simulink model "wetmodel_basic"  (R2020b)
settings: Solver=ode45  StartTime=0.0  StopTime=inf  RelTol=1e-3  EnableMultiTasking=on
libraries: dsparch4 x3, robotlib x1, dspsigops x1
settings Model: Tag=MP_system  EnablePacing=on  Creator=Andries  LastModifiedBy=LocalAdmin
settings DataIOCC: LimitDataPoints=on  SaveFormat=Array  SignalLoggingSaveFormat=ModelDataLogs  ReturnWorkspaceOutputs=off
settings OptimizationCC: ExpressionDepthLimit=2147483647  LifeSpan=inf
settings DebuggingCC: UnderspecifiedInitializationDetection=Classic  MergeDetectMultiDrivingBlocksExec=none  SolverPrmCheckMsg=warning  FcnCallInpInsideContextMsg=warning  StateNameClashWarn=warning  SFUnexpectedBacktrackingDiag=warning  SFNoUnconditionalDefaultTransitionDiag=warning  SFExecutionAtInitializationDiag=none  ArithmeticOperatorsInVariantConditions=warning
settings HardwareCC: ProdBitPerPointer=32  ProdBitPerSizeT=32  ProdBitPerPtrDiffT=32  ProdLargestAtomicFloat=None  ProdIntDivRoundTo=Undefined  ProdEndianess=Unspecified  ProdWordSize=32  ProdHWDeviceType=32-bit Generic
settings ModelReferenceCC: PropagateSignalLabelsOutOfModel=off
settings SFSimCC: SimUseLocalCustomCode=off  CustomCodeUndefinedFunction=UseInterfaceOnly
settings RTWCC: RTWUseLocalCustomCode=off
settings CodeAppCC: StateflowObjectComments=on
settings GRTTargetCC: TargetLangStandard=C89/C90 (ANSI)  CombineOutputUpdateFcns=off  GRTInterface=on
settings ConfigComp: CovMetricSettings=dw  CovSaveCumulativeToWorkspaceVar=on  CovSaveSingleToWorkspaceVar=on  CovExternalEMLEnable=off

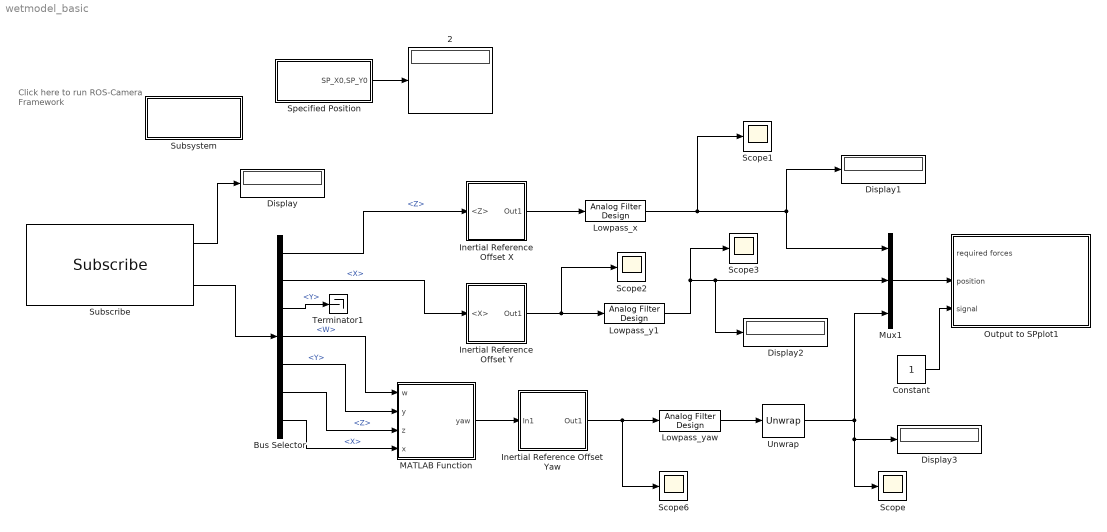
== system wetmodel_basic ==
  note: Click here to run
      | ROS-Camera Framework
  "  2" : Display
  Bus Selector : BusSelector  OutputSignals=Pose.Position.Z,Pose.Position.X,Pose.Position.Y,Pose.Orientation.W,Pose.Orientation.Y,Pose.Orientation.Z,Pose.Orientation.X
  Constant : Constant
  Display{,1..3} (4 alike) : Display
  Inertial Reference Offset X : Subsystem
  Inertial Reference Offset Y : Subsystem
  Inertial Reference Offset Yaw : Subsystem
  Lowpass_x : dsparch4/Analog Filter Design  method=Butterworth  filttype=Lowpass  N=1  Wlo=30  Whi=80  Rp=2  Rs=40
  Lowpass_y1 : dsparch4/Analog Filter Design  method=Butterworth  filttype=Lowpass  N=1  Wlo=30  Whi=80  Rp=2  Rs=40
  Lowpass_yaw : dsparch4/Analog Filter Design  method=Butterworth  filttype=Lowpass  N=8  Wlo=5  Whi=80  Rp=2  Rs=40
  MATLAB Function : MATLAB Function  TreatAsAtomicUnit=on
  Mux1 : Mux  Inputs=3
  Output to SPplot1 : Subsystem
      mask Display:
      | image(imread('spplot.JPG'))
      | port_label('input', 1, 'Req. Forces')
      | port_label('input', 2, 'Pos Update')
      | port_label('input', 3, 'signal')
  Scope{,1..3,6} (5 alike) : Scope
  Specified Position : Subsystem
  Subscribe : robotlib/Subscribe  topicSource=Select from ROS network  topic=/OptiRAS/RAS_TN_YE/pose  messageType=geometry_msgs/PoseStamped  SampleTime=-1  legacyBusStruct=off  messageQueueLength=1
  Subsystem : Subsystem  InitFcn=|  StopFcn=set_param(gcb,'BackgroundColor','red');
      | %if ros_init==1
      | if ros.internal.Global.isNodeActive == 1
      | set_param(gcb,'BackgroundColor','green');
      | else
      | set_param(gcb,'BackgroundColor','red');
      | end
      settings: ModelCloseFcn=set_param(gcb,'BackgroundColor','red');  CloseFcn=set_param(gcb,'BackgroundColor','red');
  Terminator1 : Terminator
  Unwrap : dspsigops/Unwrap  tol=pi  InputProcessing=Columns as channels (frame based)  running=off
  wires:
  Specified Position/1(SP_X0,SP_Y0) -> "  2"/1
  Mux1/1 -> Output to SPplot1/2(position)
  Subscribe/1 -> Display/1
  Constant/1 -> Output to SPplot1/3(signal)
  Subscribe/2 -> Bus Selector/1
  Lowpass_yaw/1 -> Unwrap/1
  Bus Selector/4 -> MATLAB Function/1(w)  "<W>"
  Bus Selector/5 -> MATLAB Function/2(y)  "<Y>"
  Bus Selector/6 -> MATLAB Function/3(z)  "<Z>"
  Bus Selector/7 -> MATLAB Function/4(x)  "<X>"
  Lowpass_y1/1 -> Mux1/2, Display2/1, Scope3/1
  Unwrap/1 -> Mux1/3, Scope/1, Display3/1
  Bus Selector/3 -> Terminator1/1  "<Y>"
  Inertial Reference Offset X/1(Out1) -> Lowpass_x/1
  Bus Selector/1 -> Inertial Reference Offset X/1(<Z>)  "<Z>"
  Lowpass_x/1 -> Scope1/1, Display1/1, Mux1/1
  Inertial Reference Offset Y/1(Out1) -> Scope2/1, Lowpass_y1/1
  Bus Selector/2 -> Inertial Reference Offset Y/1(<X>)  "<X>"
  Inertial Reference Offset Yaw/1(Out1) -> Lowpass_yaw/1, Scope6/1
  MATLAB Function/1(yaw) -> Inertial Reference Offset Yaw/1(In1)

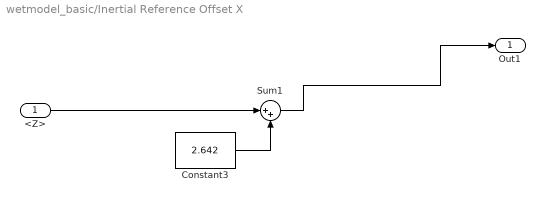
== system wetmodel_basic/Inertial Reference Offset X ==
  <Z> : Inport
  Constant3 : Constant  Value=2.642
  Sum1 : Sum  Inputs=|++
  Out1 : Outport
  wires:
  Constant3/1 -> Sum1/2
  <Z>/1 -> Sum1/1
  Sum1/1 -> Out1/1

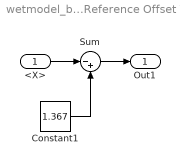
== system wetmodel_basic/Inertial Reference Offset Y ==
  <X> : Inport
  Constant1 : Constant  Value=1.367
  Sum : Sum  Inputs=|-+
  Out1 : Outport
  wires:
  Sum/1 -> Out1/1
  <X>/1 -> Sum/1
  Constant1/1 -> Sum/2

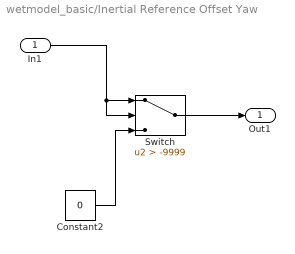
== system wetmodel_basic/Inertial Reference Offset Yaw ==
  In1 : Inport
  Constant2 : Constant  Value=0
  Switch : Switch  Criteria=u2 > Threshold  Threshold=-9999
  Out1 : Outport
  wires:
  Constant2/1 -> Switch/3
  In1/1 -> Switch/2, Switch/1
  Switch/1 -> Out1/1

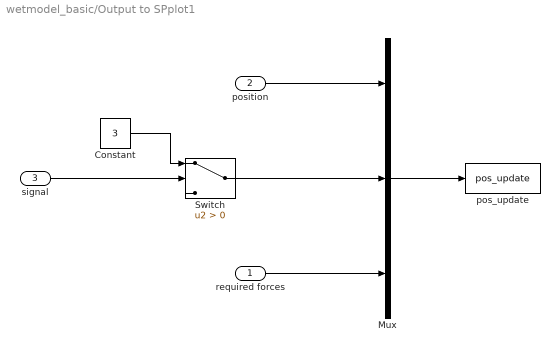
== system wetmodel_basic/Output to SPplot1 ==
  required forces : Inport
  position : Inport  Port=2
  signal : Inport  Port=3
  Constant : Constant  Value=3
  Mux : Mux  Inputs=3
  Switch : Switch  Criteria=u2 > Threshold
  pos_update : S-Function  FunctionName=pos_update  Parameters=TS_wii  SFunctionDeploymentMode=off  EnableBusSupport=off
  wires:
  Mux/1 -> pos_update/1
  position/1 -> Mux/1
  required forces/1 -> Mux/3
  Switch/1 -> Mux/2
  signal/1 -> Switch/2
  Constant/1 -> Switch/1

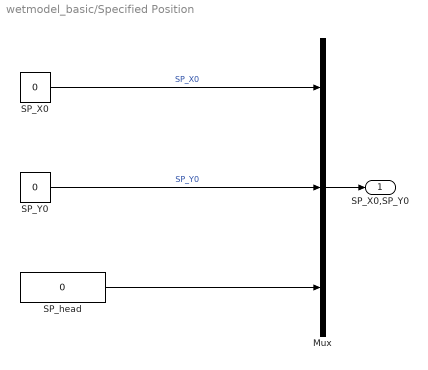
== system wetmodel_basic/Specified Position ==
  Mux : Mux  Inputs=3
  SP_X0 : Constant  Value=0
  SP_Y0 : Constant  Value=0
  SP_head : Constant  Value=0
  SP_X0,SP_Y0 : Outport
  wires:
  Mux/1 -> SP_X0,SP_Y0/1
  SP_Y0/1 -> Mux/2  "SP_Y0"
  SP_X0/1 -> Mux/1  "SP_X0"
  SP_head/1 -> Mux/3

== system wetmodel_basic/Subsystem ==

== matlab function wetmodel_basic/MATLAB Function ==
  data: w input; y input; z input; yaw output; x input
function yaw = quat2eul_VG(w,y,z,x)

%From VG MH iSCSS paper
%quatern = [ts_q4.data ts_q2.data ts_q3.data ts_q1.data]
quatern = [w,y,z,x];
%quatern = [w,x,y,z];
eulXYZ = quat2eul(quatern);
yaw = - eulXYZ(3) ;
% Change it here in case of different angle standards
